simulink subsystem "OptimalReferenceGenerator"  (R2025b)
settings: Solver=VariableStepAuto  StartTime=0.0  StopTime=10.0  RelTol=1e-3
undefined symbols (not defined in the file or in its folder): A_bar, Ts
settings Model: Creator=leeta  LastModifiedBy=leeta

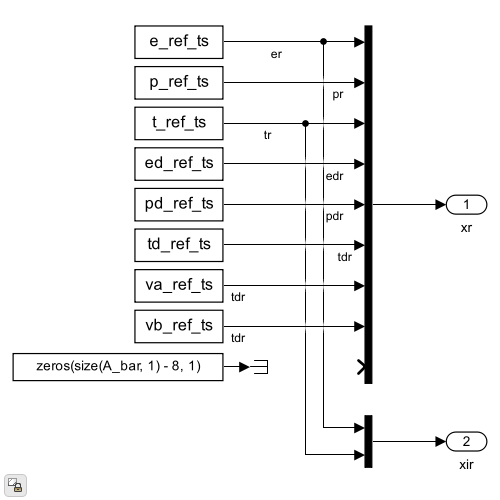
[thumbnail: Simulink's stored preview of the top-level diagram]
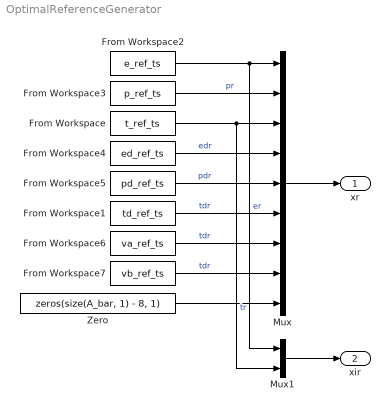
== system OptimalReferenceGenerator ==
  From Workspace : FromWorkspace  VariableName=t_ref_ts  SampleTime=Ts
  From Workspace1 : FromWorkspace  VariableName=td_ref_ts  SampleTime=Ts
  From Workspace2 : FromWorkspace  VariableName=e_ref_ts  SampleTime=Ts
  From Workspace3 : FromWorkspace  VariableName=p_ref_ts  SampleTime=Ts
  From Workspace4 : FromWorkspace  VariableName=ed_ref_ts  SampleTime=Ts
  From Workspace5 : FromWorkspace  VariableName=pd_ref_ts  SampleTime=Ts
  From Workspace6 : FromWorkspace  VariableName=va_ref_ts  SampleTime=Ts
  From Workspace7 : FromWorkspace  VariableName=vb_ref_ts  SampleTime=Ts
  Mux : Mux  Inputs=9
  Mux1 : Mux  Inputs=2
  Zero : Constant  Value=zeros(size(A_bar, 1) - 8, 1)
  xr : Outport
  xir : Outport  Port=2
  wires:
  Mux/1 -> xr/1
  From Workspace/1 -> Mux/3, Mux1/2  "tr"
  From Workspace2/1 -> Mux/1, Mux1/1  "er"
  From Workspace1/1 -> Mux/6  "tdr"
  Mux1/1 -> xir/1
  From Workspace3/1 -> Mux/2  "pr"
  From Workspace4/1 -> Mux/4  "edr"
  From Workspace5/1 -> Mux/5  "pdr"
  From Workspace6/1 -> Mux/7  "tdr"
  From Workspace7/1 -> Mux/8  "tdr"
  Zero/1 -> Mux/9
